simulink model "MARCH_v1_6"  (R2016a)
settings: Solver=FixedStepDiscrete  StartTime=0.0  StopTime=inf  FixedStep=0.001  RelTol=1e-3
InitFcn:
  | cd(fileparts(which(bdroot)));
  | 
  | init_model
  | initialize_model_testingBlocks
StartFcn:
  | cd(fileparts(which(bdroot)));
StopFcn:
  | cd(fileparts(which(bdroot)));
model workspace (MAT data in the model file):
  localValue = 1
  targetValue = 1
undefined symbols (not defined in the file or in its folder): Hip_HAA, Left_Leg, Right_Leg
libraries: xpcethercatlib x56, slrtlib x8, simulink x1, dspnetwork x1, aerolibanimutils x1
(part 2 of 2)

== system MARCH_v1_6/Input Device/Generate random block signal safety/Create peak2 ==
  In1 : Inport
  Delay : Delay  DelayLength=1
  Greater than 0 : MATLAB Function  TreatAsAtomicUnit=on
  Sum : Sum  Inputs=|-+
  Out1 : Outport
  wires:
  Sum/1 -> Greater than 0/1(peak)
  In1/1 -> Sum/2, Delay/1
  Delay/1 -> Sum/1
  Greater than 0/1(signal) -> Out1/1

== system MARCH_v1_6/Input Device/Generate random block signal safety/Create peak3 ==
  In1 : Inport
  Delay : Delay  DelayLength=1
  Greater than 0 : MATLAB Function  TreatAsAtomicUnit=on
  Sum : Sum  Inputs=|-+
  Out1 : Outport
  wires:
  Sum/1 -> Greater than 0/1(peak)
  In1/1 -> Sum/2, Delay/1
  Delay/1 -> Sum/1
  Greater than 0/1(signal) -> Out1/1

== system MARCH_v1_6/Input Device/Generate random block signal trigger/Create peak1 ==
  In1 : Inport
  Delay : Delay  DelayLength=1
  Greater than 0 : MATLAB Function  TreatAsAtomicUnit=on
  Sum : Sum  Inputs=|-+
  Out1 : Outport
  wires:
  Sum/1 -> Greater than 0/1(peak)
  In1/1 -> Sum/2, Delay/1
  Delay/1 -> Sum/1
  Greater than 0/1(signal) -> Out1/1

== system MARCH_v1_6/Input Device/Generate random block signal trigger/Create peak2 ==
  In1 : Inport
  Delay : Delay  DelayLength=1
  Greater than 0 : MATLAB Function  TreatAsAtomicUnit=on
  Sum : Sum  Inputs=|-+
  Out1 : Outport
  wires:
  Sum/1 -> Greater than 0/1(peak)
  In1/1 -> Sum/2, Delay/1
  Delay/1 -> Sum/1
  Greater than 0/1(signal) -> Out1/1

== system MARCH_v1_6/Input Device/Generate random block signal trigger/Create peak3 ==
  In1 : Inport
  Delay : Delay  DelayLength=1
  Greater than 0 : MATLAB Function  TreatAsAtomicUnit=on
  Sum : Sum  Inputs=|-+
  Out1 : Outport
  wires:
  Sum/1 -> Greater than 0/1(peak)
  In1/1 -> Sum/2, Delay/1
  Delay/1 -> Sum/1
  Greater than 0/1(signal) -> Out1/1

== matlab function MARCH_v1_6/Reachability/MATLAB Function ==
  data: q input size=6; q_out output size=6; err output size=6
function [q_out, err] = fcn(q)

joint_limit_min = [-20 -109 -3 -23 -109 -3]'/180*pi;
joint_limit_max = [23 21 121 20 21 121]'/180*pi;

n = size(q,2);
%% Check if all joints are within limits

err = imag(q)~=0 | q<repmat(joint_limit_min,n,1) | q>repmat(joint_limit_max,n,1);
q_out = q;

== matlab function MARCH_v1_6/Controllers/Continuous Gait/Trajectory ==
  data: stepHeight input; q output; done output; stepLength input; q input size=[1 6]; torso_z output; debugIn input; base output; debug output
function [q,done, torso_z, base, debug]= fcn(stepHeight,stepLength,q,debugIn)
%#codegen

persistent r splineCtrl i trajectory fullStep fullWeightShift torsoTrajectory;

%% Initialize all variables
if(isempty(splineCtrl))
    splineCtrl = splineController();
end

if(isempty(fullStep))
    fullStep = 0;
    fullWeightShift = 0;
end

if(isempty(r))
    % Get frequency of the model
    r = robotics();
    r.base = 1;
    
end

if(isempty(i))
    i = 0;
end

if(isempty(trajectory))
    trajectory = [];
    torsoTrajectory = [];
end

%% Logic
% Only run this for the beginning of the swing
r.setTorsoHeight(debugIn);
if(~i)
    
    
    % We set the method of whether we want an analytically generated spline
    % or a spline directly from the database.
    % Options: 'circle' and 'stairs'
    splineCtrl.setStepLength(stepLength).setStepHeight(stepHeight);
    if(~fullStep)
        trajectory = splineCtrl.method('circle').setVelocity(0.7).getHalfStep();
        fullStep = 1;
    else
        trajectory = splineCtrl.method('circle').setVelocity(0.7).getFullStep();
    end
    
    % Transform the spline to the correct frame based on which foot is
    % swinging
    trajectory = r.transformSpline(trajectory);
    
    
    torso_delta = [0 0.1 0];
    
    % Weight shift to base foot
    if(r.base == 1)
        torso_delta(2) = abs(torso_delta(2));
    else
        torso_delta(2) = -abs(torso_delta(2));
    end
    
    if(~fullWeightShift)
        torsoTrajectory = splineCtrl.getHalfWeightShift(torso_delta);
        fullWeightShift = 1;
    else
        torsoTrajectory = splineCtrl.getFullWeightShift(torso_delta);
    end
    
    i = i+1;
end

r.point = [trajectory(1,i) trajectory(2,i) trajectory(3,i)];
debug = r.point;
r.step();
r.weightShift(torsoTrajectory(i,:));

r.inverseKinematics();
q = r.q;

torso_z = r.torso_z;

% Set final values as initial values for the next iteration
r.refresh();

% Reset iterator after we're done with the trajectory, otherwise we
% increment the counter and continue iterating as simulink continues
% sampling
if( i < (length(trajectory)))
    i = i+1;
    done = 0;
else
    i = 0;
    r.switchFoot(r.base);
    done = 1;
end

% Output which foot is currently ON THE GROUND
base = r.base;
end

== matlab function MARCH_v1_6/Controllers/Continuous Gait/Torso Trajectory ==
  data: desired input; current input; z output
function z = fcn(desired, current)
%#codegen

persistent trajectory i desiredPersistent;

% Speed at which we home in SAMPLES
samples = 1000;

if (isempty(i))
    i = 0;
    
    % Hack to fix initial condition of delay during init phase
    current = desired;
end

if(isempty(desiredPersistent))
    desiredPersistent = desired;
end

if(isempty(trajectory))
    trajectory = linspace(current,desiredPersistent,samples);
end

if(desiredPersistent ~= desired)
    trajectory = linspace(current,desired,samples);
    desiredPersistent = desired;
    i = 0;
end

if(i < samples)
    i = i+1;
end

z = trajectory(i);

== matlab function MARCH_v1_6/Controllers/Switcher ==
  data: index output; i input; enable output
function [index, enable]= fcn(i)
%#codegen

% This function is supposed to take a state and switch between controllers.
% Currently it directly routes the input argument as the index. In the
% future this can be something different so I have left it open for
% future modifications.

% The u vector represents the controllers. When the vector consists out of
% zeros it will not enable any controller. In the case that an index is set
% to a non zero value, the controller which belongs to that index will be
% enabled.
u = zeros(10,1);

u(i) = 2;

index = i;
enable = u;

== matlab function MARCH_v1_6/EtherCAT Joint Data In/MATLAB Function ==
  data: encoderValue input; angles output; par parameter
function angles = convertToJointAngles(encoderValue, par)
angles = zeros(6,1);

for i = 1:6
    angles(i) = enc2rad(encoderValue(i), i, par);
end

== matlab function MARCH_v1_6/Controllers/Walking/Trajectory ==
  data: base input; q output; done output; action input; stepType input; q input size=[1 6]
function [q,done]= fcn(base,action,stepType, q)
%#codegen

persistent r splineCtrl i triggerPersistent torsoTrajectory trajectory hold fullWeightShift;

%% Initialize all variables
if(isempty(splineCtrl))
    splineCtrl = splineController();
end

if(isempty(fullWeightShift))
    fullWeightShift = 0;
end

if(isempty(stepType))
    stepType = 0;
end

if(isempty(r))
    % Get frequency of the model
    r = robotics();
    r.base = base;
    
end

if(isempty(hold))
    hold = 0;
end

if(isempty(i))
    i = 0;
end

if(isempty(triggerPersistent))
    triggerPersistent = action;
end


if(isempty(trajectory))
    trajectory = [0 0 0];
    torsoTrajectory = [0 0 0];
end

%% Logic
% Only run this for the beginning of the swing
done = 0;

% Reset values if trigger is toggled.
if(triggerPersistent ~= action)
    r.base = base;
    i = 0;
    hold = 0;
    triggerPersistent = action;
end

% Hold exoskeleton in same position after a single step
if(hold)
    q = r.q;
    done = 1;
    return
end

if(~i)
    % Foot Trajectory
    splineCtrl.setStepHeight(0.5).setStepLength(0.5);
    if(~stepType)
        trajectory = splineCtrl.method('circle').setVelocity(0.5).getHalfStep();
    else
        trajectory = splineCtrl.method('circle').setVelocity(0.5).getFullStep();
    end
    
    trajectory = r.transformSpline(trajectory);
    
    % Weight shift to base foot
    torso_delta = [0 0.07 0];
    
    if(r.base == 1)
        torso_delta(2) = abs(torso_delta(2));
    else
        torso_delta(2) = -abs(torso_delta(2));
    end
    
    if(~stepType)
        torsoTrajectory = splineCtrl.getHalfWeightShift(torso_delta);
    else
        torsoTrajectory = splineCtrl.getFullWeightShift(torso_delta);
    end
    
    
    i = i+1;
end

r.point = [trajectory(1,i) trajectory(2,i) trajectory(3,i)];
r.step();
r.weightShift(torsoTrajectory(i,:));
r.inverseKinematics();

q = r.q;

% Set final values as initial values for the next iteration
r.refresh();

% Reset iterator after we're done with the trajectory, otherwise we
% increment the counter and continue iterating as simulink continues
% sampling
if( i < (length(trajectory)))
    i = i+1;
else
    hold = 1;
end

end

== matlab function MARCH_v1_6/Controllers/Hold/MATLAB Function ==
  data: q_in input size=[1 6]; q_out output double size=[1 6]; reset input
function q_out = fcn(q_in,reset)
persistent q_hold hold

if(isempty(q_hold))
   q_hold = zeros(1,6); 
   hold = 0;
end

if(reset)
   hold = 0; 
end

if(~hold)
    q_hold = q_in;
    hold = 1;
end

q_out = q_hold;

== matlab function MARCH_v1_6/Input Device/Generate random block signal safety/Create peak1/Greater than 0 ==
  data: peak input; signal output
function signal  = fcn(peak)


if peak >= 0
    signal = peak;
else
    signal = 0;
    
    
end

== matlab function MARCH_v1_6/State Machine/Create peak3/Greater than 0 ==
  data: peak input; signal output
function signal  = fcn(peak)


if peak >= 0
    signal = peak;
else
    signal = 0;
    
    
end

== matlab function MARCH_v1_6/Controllers/Point & Go/Trajectory ==
  data: base input; q output; action input; point input; q input size=[1 6]; debugOut output; debugIn input
function [q,debugOut]= fcn(base,action, point,q,debugIn)
%#codegen

persistent r splineCtrl i triggerPersistent trajectory fullStep hold pointPersistent;

%% Initialize all variables
if(isempty(splineCtrl))
    splineCtrl = splineController();
end


if(isempty(fullStep))
    fullStep = 0;
end

if(isempty(r))
    r = robotics();
    r.base = base;
    
end

if(isempty(hold))
    hold = 0;
end

if(isempty(i))
    i = 0;
end

if(isempty(triggerPersistent))
    triggerPersistent = action;
end

if(isempty(pointPersistent))
    pointPersistent = point;
end

if(isempty(trajectory))
    trajectory = [0 0];
end

%% Logic

% Reset values if trigger is toggled.
if(triggerPersistent ~= action)
    r.base = base;
    i = 0;
    hold = 0;
    triggerPersistent = action;
end


% Hold exoskeleton in same position after a single step
if(hold)
    debugOut = r.torso_z;
    q = r.q;
    return
end

if(~i)
    
    % We set the method of whether we want an analytically generated spline
    % or a spline directly from the database.
    % Options: 'circle' and 'stairs'
    splineCtrl.setStepHeight(0.3);
    trajectory = splineCtrl.method('circle').getStepFromPoint(point);
    
    
    
    % Transform the spline to the correct frame based on which foot is
    % swinging
    trajectory = r.transformSpline(trajectory);
    
    i = i+1;
end

r.point = [trajectory(1,i) trajectory(2,i) trajectory(3,i)];

r.stepPosture();
r.inverseKinematics();

q = r.q;
debugOut = r.torso_z;

% Set final values as initial values for the next iteration
r.refresh();

% Reset iterator after we're done with the trajectory, otherwise we
% increment the counter and continue iterating as simulink continues
% sampling
if( i < (length(trajectory)))
    i = i+1;
else
    hold = 1;
end

end

== matlab function MARCH_v1_6/State Machine/Input Interpreter Safety ==
  data: rightIn input; rightOut output; leftIn input; leftOut output; bothOut output
function [rightOut, leftOut, bothOut]= fcn(rightIn, leftIn)

persistent countRight countLeft countBoth

if (isempty(countRight)||isempty(countLeft)||isempty(countBoth));
    countRight = 0;
    countLeft = 0;
    countBoth = 0;
    rightOut = 0;
    leftOut = 0;
    bothOut = 0;
end

threshold = 700;


if (rightIn == 0 && leftIn == 0)
    rightOut = 0;
    leftOut = 0;
    bothOut = 0;
    countRight = 0;
    countLeft = 0;
    countBoth = 0;
elseif (rightIn == 1 && leftIn ~= 1)
    countRight = countRight + 1;
    countLeft = 0;
    countBoth = 0;
    if countRight == threshold
        rightOut = 1;
        leftOut = 0;
        bothOut = 0;
        countRight = 0;
    else
        rightOut = 0;
        leftOut = 0;
        bothOut = 0;
    end
elseif (leftIn == 1 && rightIn ~= 1)
    countRight = 0;
    countLeft = countLeft + 1;
    countBoth = 0;
    if countLeft == threshold
        rightOut = 0;
        leftOut = 1;
        bothOut = 0;
        countLeft = 0;
    else
        rightOut = 0;
        leftOut = 0;
        bothOut = 0;
    end
elseif (rightIn == 1 && leftIn == 1)
    countRight = 0;
    countLeft = 0;
    countBoth = countBoth + 1;
    if countBoth == threshold
        rightOut = 0;
        leftOut = 0;
        bothOut = 1;
    else
        rightOut = 0;
        leftOut = 0;
        bothOut = 0;
    end
else
    rightOut = -1;
    leftOut = -1;
    bothOut = -1;
end

== matlab function MARCH_v1_6/EtherCAT Joint Setpoints/exoskeleton/MATLAB Function ==
  data: jointAngle input; encVal output; par parameter
function encVal = convertToEncoderValues(jointAngle, par)
encVal = zeros(6,1);

for i = 1:6
    encVal(i) = rad2enc(jointAngle(i), i, par);
end

== matlab function MARCH_v1_6/Controllers/StandUp/Trajectory ==
  data: done output; q output; action input; q_i input size=[1 6]; debugIn input
function [done,q] = fcn(action,q_i,debugIn)
%#codegen

persistent r splineCtrl i q_t;

%% Initialize all variables
if(isempty(splineCtrl))
    splineCtrl = splineController();
end

if(isempty(r))
    % Get frequency of the model
    r = robotics();
    
end

if(isempty(q_t))
   q_t = [0 0 0 0 0 0];
end

if(isempty(i))
    i = 0;
end


%% Logic
done = 0;
if(~i)
    % Calculate final position based on robotics parameters
    r.setTorsoHeight(r.torso_z);
    r.refresh();
    r.inverseKinematics();
    q_f = r.q;
    
    splineCtrl.samples = 4000;
    q_t = splineCtrl.getStandupJointTrajectory(q_i,q_f);
    
%     q_t = splineCtrl.ease(q_t);
    
    i = i+1;
end

q = q_t(i,:);

if( i < length(q_t))
    i = i+1;
else
   done = 1; 
end

end

== matlab function MARCH_v1_6/State Machine/Input Interpreter Triggers ==
  data: rightIn input; rightOut output; leftIn input; leftOut output; bothOut output
function [rightOut, leftOut, bothOut]= fcn(rightIn, leftIn)

persistent countRight countLeft countBoth

if (isempty(countRight)||isempty(countLeft)||isempty(countBoth));
    countRight = 0;
    countLeft = 0;
    countBoth = 0;
    rightOut = 0;
    leftOut = 0;
    bothOut = 0;
end

threshold = 700;


if (rightIn == 0 && leftIn == 0)
    rightOut = 0;
    leftOut = 0;
    bothOut = 0;
    countRight = 0;
    countLeft = 0;
    countBoth = 0;
elseif (rightIn == 1 && leftIn ~= 1)
    countRight = countRight + 1;
    countLeft = 0;
    countBoth = 0;
    if countRight == threshold
        rightOut = 1;
        leftOut = 0;
        bothOut = 0;
        countRight = 0;
    else
        rightOut = 0;
        leftOut = 0;
        bothOut = 0;
    end
elseif (leftIn == 1 && rightIn ~= 1)
    countRight = 0;
    countLeft = countLeft + 1;
    countBoth = 0;
    if countLeft == threshold
        rightOut = 0;
        leftOut = 1;
        bothOut = 0;
        countLeft = 0;
    else
        rightOut = 0;
        leftOut = 0;
        bothOut = 0;
    end
elseif (rightIn == 1 && leftIn == 1)
    countRight = 0;
    countLeft = 0;
    countBoth = countBoth + 1;
    if countBoth == threshold
        rightOut = 0;
        leftOut = 0;
        bothOut = 1;
    else
        rightOut = 0;
        leftOut = 0;
        bothOut = 0;
    end
else
    rightOut = -1;
    leftOut = -1;
    bothOut = -1;
end

== matlab function MARCH_v1_6/Controllers/Stairs/Torso Trajectory ==
  data: desired input; torsoTrajectory output size=[1 3]
function torsoTrajectory = fcn(desired)
%#codegen

persistent trajectory i desiredPersistent;

% Speed at which we home in SAMPLES
samples = 1000;

if (isempty(i))
    i = 0;
end

if(isempty(desiredPersistent))
    desiredPersistent = desired;
end

if(isempty(trajectory))   
    desiredPersistent = desired;
    
    trajectory = [linspace(0,desiredPersistent(1),samples)
        linspace(0,desiredPersistent(2),samples)
        linspace(0,desiredPersistent(3),samples) ]';
end

if(~isequal(desiredPersistent,desired))
    trajectory = [linspace(0,desired(1),samples)
        linspace(0,desired(2),samples)
        linspace(0,desired(3),samples) ]';
    
    desiredPersistent = desired;
    i = 0;
end

if(i < samples)
    i = i+1;
end

torsoTrajectory = trajectory(i,:);

== matlab function MARCH_v1_6/Controllers/Stairs/Trajectory ==
  data: base input; q output; action_t input; q input size=[1 6]; torso_delta input size=[1 3]
function q  = fcn(base,action_t,q,torso_delta)
%#codegen

persistent r s i j trigger trajectory torsoTrajectory seq;

%% Initialize all variables
if(isempty(s))
    s = splineController();
end

if(isempty(r))
    % Get frequency of the model
    r = robotics();
    r.base = base;
    
end

if(isempty(seq))
    seq = 1;
end

if(isempty(i) || isempty(j))
    i = 0;
    j = 0;
end

if(isempty(trigger))
    trigger = action_t;
end

if(isempty(torsoTrajectory))
    torsoTrajectory = [0 0 0];
end

if(isempty(trajectory))
    trajectory = [0 0 0];
end

%% Weight shifting sequence
% This sequence will weight shift to the base leg. The entire sequence is
% wrapped inside an if statement to prevent this from executing after it
% has been completed. It is either this or a separate function block which
% would be a disaster because the classes are separate instances.
if(seq == 1)
    if (~i)
        r.setTorsoHeight(0.95);
        r.refresh(); % make sure initial position of torso has same heighit as set above
        % Override sample speed
        s.samples = 1000;
        
        % Weight shift to base foot
        if(base == 1)
            torso_delta(2) = -abs(torso_delta(2));
        else
            torso_delta(2) = abs(torso_delta(2));
        end
        
        torsoTrajectory = s.getHalfWeightShift(torso_delta);
        i = i+1;
    end
    
    % Playback trajectory and return preventing doing the rest
    if(i < length(torsoTrajectory))
        r.reset();
        r.weightShift(torsoTrajectory(i,:));
        r.inverseKinematics();
        q = r.q;
        
        i = i+1;
        return
    else
        q = r.q;
        
        % Init and enable step sequence
        r.refresh();
        j = 0;
        % Disable weight shifting
        seq = 2;
    end
end

%% Step Sequence
% This sequence will step onto the stair
if(seq == 2)
    if(~j)
        s.setStepHeight(0.2).setStepLength(0.5);
        
        trajectory = s.method('circle').setVelocity(0.21).getHalfStep();
        trajectory = r.transformSpline(trajectory);
        if(r.base == 1)
            torso_delta(2) = -abs(torso_delta(2));
        else
            torso_delta(2) = abs(torso_delta(2));
        end
        % Shift the weight back to the middle during the step
        torsoTrajectory = s.getWeightShift(torso_delta, [0 0 0]);
        
        j = j+1;
    end
    
    r.point = [trajectory(1,j) trajectory(2,j) trajectory(3,j)];
    r.step();

    % Weight shift the torso back to the middle
    r.weightShift(torsoTrajectory(j,:));
    r.inverseKinematics();
    
    q = r.q;
    
    % THIS SHOULD NOT BE HERE BUT IT WON'T WORK OTHERWISE :(
    r.refresh();
    
    if(j < length(trajectory))
        j = j+1;
    else
        j = 0;
        q = r.q;
        r.switchFoot(r.base);
    end
    
end
end

== matlab function MARCH_v1_6/Controllers/0-Torque/RHFE/Sample and Hold ==
  data: offset input; reference output
function reference = fcn(offset)
%#codegen

persistent offsetPersistent hold;

if(isempty(offsetPersistent))
    offsetPersistent = int32(0);
    hold = 0;
end

if(offset > 0 && hold == 0)
    
    offsetPersistent = offset;
    hold = 1;
end

reference = offsetPersistent;

== stateflow chart MARCH_v1_6/State Machine/State Machine ==
  state InputDeviceCheck
    en: controllerIndex = 1;
    en: action = 0;
    en: base = 0;
    en: stepType = 0;
    en: state = 0;
    state checkScrollClick
      en: inpDevWorking = 0;
    state checkBothSafety
      en: inpDevWorking = 0;
    state checkbothTrigger
      en: inpDevWorking = 0;
    state InpDev
      en: inpDevWorking = 1;
    (default) -> checkScrollClick : [rightScrollMode == 1]
    checkScrollClick -> checkBothSafety [order 1] : [rightScrollClick == 1]
    checkBothSafety -> checkbothTrigger : [bothSafety == 1]
    checkbothTrigger -> InpDev : [bothTriggers == 1]
  state ZeroTorque
    en: controllerIndex = 1;
    en: action = 0;
    en: base = 0;
    en: stepType = 0;
    en: state = 1;
  state testingBypass
    en: controllerIndex = 1;
    en: action = 0;
    en: base = 0;
    en: stepType = 0;
    en: state = 9;
  state SitDown
    en: controllerIndex = 4;
    en: action = 0;
    en: base = 0;
    en: stepType = 0;
    en: state = 4;
  state HoldPosition
    en: controllerIndex = 2;
    en: action = 0;
    en: base = 0;
    en: stepType = 0;
    en: state = 2;
  state StandUp
    en: controllerIndex = 3;
    en: action = 0;
    en: base = 0;
    en: stepType = 0;
    en: state = 3;
  state DiscreteGait
    en: controllerIndex = 5;
    state standbyModeDiscr
      en: action = actionLocal;
      en: base = baseLocal;
      en: stepType = 0;
      en: state = 61;
      % satandby mode from discrete gait
      % exoskeleton finishes full step, makes complementary halfstep, then stands still
    state makeLeftHalfStepDiscr
      en: action = action+1;
      en: base = 1;
      en: stepType = 0;
      en: state = 61;
      baseLocal = base;
      actionLocal = action;
    state makeRightHalfStepDiscr
      en: action = action+1;
      en: base = 3;
      en: stepType = 0;
      en: state = 61;
      baseLocal = base;
      actionLocal = action;
    state startLeftHalfStepDiscr
      en: action = 1;
      en: base = 1;
      en: stepType = 0;
      en: state = 6;
      baseLocal = base
    state finishRightFullStepDiscr
      en: action = actionLocal;
      en: base = 3;
      en: stepType = 1;
      en: state = 61;
      baseLocal = base;
      % exoskeleton finishes right full step
    state finishLeftFullStepDiscr
      en: action = actionLocal;
      en: base = 1;
      en: stepType = 1;
      en: state = 61;
      baseLocal = base;
      % exoskeleton finishes left full step
    state makeLeftHalfStepDiscr1
      en: action = action+1;
      en: base = 1;
      en: stepType = 0;
      en: state = 62;
      baseLocal = base;
      actionLocal = action;
    state makeRightHalfStepDiscr3
      en: action = action+1;
      en: base = 3;
      en: stepType = 0;
      en: state = 62;
      baseLocal = base;
      actionLocal = action;
    state leftFullStepDiscr
      en: action = action+1;
      en: base = 1;
      en: stepType = 1;
      en: state = 6;
      baseLocal = base;
      actionLocal = action;
    state rightFullStepDiscr
      en: action = action+1;
      en: base = 3;
      en: stepType = 1;
      en: state = 6;
      baseLocal = base;
      actionLocal = action;
    state safeDiscr2Walk1
      en: action = actionLocal;
      en: base = baseLocal;
      en: stepType = 1;
      en: state = 62;
    state safeDiscr2Walk
      en: action = actionLocal;
      en: base = baseLocal;
      en: stepType = 1;
      en: state = 62;
    state safeModeDiscr
      en: action = actionLocal;
      en: base = baseLocal;
      en: stepType = 1;
      en: state = 62;
      % safemode from discr. gait
      % exoskeleton finishes full step, then stands still
    makeRightHalfStepDiscr3 -> standbyModeDiscr : [done == 1]
    makeLeftHalfStepDiscr1 -> standbyModeDiscr : [done == 1]
    standbyModeDiscr -> startLeftHalfStepDiscr [order 2] : [bothTriggers == 1]
    makeLeftHalfStepDiscr -> standbyModeDiscr : [done == 1]
    makeRightHalfStepDiscr -> standbyModeDiscr : [done == 1]
    finishLeftFullStepDiscr -> makeRightHalfStepDiscr : [done == 1]
    finishRightFullStepDiscr -> makeLeftHalfStepDiscr : [done == 1]
    startLeftHalfStepDiscr -> rightFullStepDiscr : [done == 1 && rightTrigger == 1]
    leftFullStepDiscr -> finishLeftFullStepDiscr [order 1] : [bothTriggers == 1]
    rightFullStepDiscr -> finishRightFullStepDiscr [order 1] : [bothTriggers == 1]
    (junction 178) -> makeRightHalfStepDiscr3 [order 2] : [baseLocal == 1]
    (junction 178) -> makeLeftHalfStepDiscr1 [order 1] : [baseLocal == 3]
    rightFullStepDiscr -> leftFullStepDiscr [order 2] : [done == 1 && leftTrigger ==  1]
    leftFullStepDiscr -> rightFullStepDiscr [order 2] : [done == 1 && rightTrigger == 1]
    safeDiscr2Walk1 -> leftFullStepDiscr [order 2] : [leftTrigger == 1 && baseLocal == 3]
    leftFullStepDiscr -> safeModeDiscr [order 3] : [bothSafety == 1]
    rightFullStepDiscr -> safeModeDiscr [order 3] : [bothSafety == 1]
    safeDiscr2Walk1 -> rightFullStepDiscr [order 1] : [rightTrigger == 1 && baseLocal == 1]
    safeDiscr2Walk -> safeDiscr2Walk1 : [done == 1]
    safeModeDiscr -> safeDiscr2Walk [order 1] : [bothSafety == 1]
    safeModeDiscr -> (junction 178) [order 2] : [bothTriggers == 1 && done == 1]
  state ContinuousGait
    en: controllerIndex = 5;
    state standbyModeCont
      en: action = actionLocal;
      en: base = baseLocal;
      en: stepType = 0;
      en: state = 51;
      % satandby mode from continuous gait
      % exoskeleton finishes full step, makes complementary halfstep, then stands still
    state makeLeftHalfStepCont
      en: action = action+1
      en: base = 1;
      en: stepType = 0;
      en: state = 51;
      baseLocal = base;
    state makeRightHalfStepCont
      en: action = action+1;
      en: base = 3;
      en: stepType = 0;
      en: state = 51;
      baseLocal = base;
      actionLocal = action;
    state startLeftHalfStepCont
      en: action = 1;
      en: base = 1;
      en: stepType = 0;
      en: state = 5;
      baseLocal = base
    state finishLeftFullStepCont
      en: action = actionLocal;
      en: base = 1;
      en: stepType = 1;
      en: state = 51;
      baseLocal = base;
      % exoskeleton finishes left full step
    state finishRightFullStepCont
      en: action = actionLocal
      en: base = 3;
      en: stepType = 1;
      en: state = 51;
      baseLocal = base;
      % exoskeleton finishes right full step
    state makeRightHalfStepCont1
      en: action = action+1;
      en: base = 3;
      en: stepType = 0;
      en: state = 52;
      baseLocal = base;
      actionLocal = action;
    state makeLeftHalfStepCont1
      en: action = action+1;
      en: base = 1;
      en: stepType = 0;
      en: state = 52;
      baseLocal = base;
      actionLocal = action
    state leftFullStepCont
      en: action = action+1;
      en: base = 1;
      en: stepType = 1;
      en: state = 5;
      baseLocal = base;
      actionLocal = action;
    state rightFullStepCont
      en: action = action+1
      en: base = 3;
      en: stepType = 1;
      en: state = 5;
      baseLocal = base;
      actionLocal = action;
    state safeCont2Walk
      en: action = actionLocal;
      en: base = baseLocal;
      en: stepType = 1;
      en: state = 52;
    state safeModeCont
      en: action = actionLocal;
      en: base = baseLocal;
      en: stepType = 1;
      en: state = 52;
      % safemode from cont. gait
      % exoskeleton finishes full step, then stands still
    makeRightHalfStepCont1 -> standbyModeCont : [done == 1]
    standbyModeCont -> startLeftHalfStepCont [order 2] : [bothTriggers == 1]
    makeLeftHalfStepCont1 -> standbyModeCont : [done == 1]
    makeRightHalfStepCont -> standbyModeCont : [done == 1]
    makeLeftHalfStepCont -> standbyModeCont : [done == 1]
    finishLeftFullStepCont -> makeRightHalfStepCont : [done == 1]
    finishRightFullStepCont -> makeLeftHalfStepCont : [done == 1]
    startLeftHalfStepCont -> rightFullStepCont : [done == 1]
    leftFullStepCont -> finishLeftFullStepCont [order 2] : [bothTriggers == 1]
    rightFullStepCont -> finishRightFullStepCont [order 1] : [bothTriggers == 1]
    (junction 172) -> makeRightHalfStepCont1 [order 2] : [baseLocal == 1]
    (junction 172) -> makeLeftHalfStepCont1 [order 1] : [baseLocal == 3]
    leftFullStepCont -> rightFullStepCont [order 3] : [done == 1]
    rightFullStepCont -> leftFullStepCont [order 3] : [done == 1]
    safeCont2Walk -> rightFullStepCont [order 1] : [done == 1 && baseLocal == 1]
    rightFullStepCont -> safeModeCont [order 2] : [bothSafety == 1]
    safeCont2Walk -> leftFullStepCont [order 2] : [done == 1 && baseLocal == 3]
    leftFullStepCont -> safeModeCont [order 1] : [bothSafety == 1]
    safeModeCont -> safeCont2Walk [order 1] : [bothSafety == 1]
    safeModeCont -> (junction 172) [order 2] : [bothTriggers == 1 && done == 1]
  (default) -> InputDeviceCheck : [rightScrollMode == 0]
  checkScrollClick -> testingBypass [order 2] : [rightScrollMode == 9]
  InputDeviceCheck -> ZeroTorque : [inpDevWorking == 1]
  ZeroTorque -> HoldPosition : [rightScrollMode == 3 && rightScrollClick == 1]
  SitDown -> ZeroTorque [order 1] : [rightScrollMode == 1 && rightScrollClick == 1 && done == 1]
  HoldPosition -> ZeroTorque [order 1] : [rightScrollMode == 1 && rightScrollClick == 1]
  testingBypass -> StandUp : [rightScrollClick == 1]
  SitDown -> StandUp [order 2] : [rightScrollMode == 3 && rightScrollClick == 1 && done == 1]
  StandUp -> SitDown [order 3] : [rightScrollMode ==4 && rightScrollClick == 1 && done == 1]
  HoldPosition -> StandUp [order 2] : [rightScrollMode == 3 && bothTriggers == 1]
  standbyModeCont -> StandUp [order 1] : [rightScrollMode == 3 && rightScrollClick == 1]
  StandUp -> startLeftHalfStepCont [order 2] : [rightScrollMode == 5 && rightScrollClick == 1 && done == 1]
  StandUp -> startLeftHalfStepDiscr [order 1] : [rightScrollMode == 6 && rightScrollClick == 1 && done == 1]
  standbyModeDiscr -> StandUp [order 1] : [rightScrollMode == 3 && rightScrollClick == 1]
  data: rightTrigger input; leftTrigger input; bothTriggers input; rightSafety input; leftSafety input; bothSafety input; rightScrollMode input; rightScrollClick input; controllerIndex output; action output; base output; inpDevWorking local; done input; stepType output; state output; baseLocal local; actionLocal local

== matlab function MARCH_v1_6/Input Device/Generate random block signal safety/Create peak2/Greater than 0 ==
  data: peak input; signal output
function signal  = fcn(peak)


if peak >= 0
    signal = peak;
else
    signal = 0;
    
    
end

== matlab function MARCH_v1_6/Input Device/Generate random block signal safety/Create peak3/Greater than 0 ==
  data: peak input; signal output
function signal  = fcn(peak)


if peak >= 0
    signal = peak;
else
    signal = 0;
    
    
end

== matlab function MARCH_v1_6/Input Device/Generate random block signal safety/Rand. Block Func. Gen.1 ==
  data: u input; delayDurationInp input; blockDurationInp input; output output
function output  = fcn(u, delayDurationInp, blockDurationInp)

%% initialize the variable
persistent delayDuration blockDuration

if(isempty(blockDuration)||isempty(delayDuration))
    blockDuration = 0;
    delayDuration = 0;
    output = 0;
end

%% check if the delay and the block are done

doneDelay = (delayDuration <= 0);
doneBlock = (blockDuration <= 0);
done = (doneDelay && doneBlock);



%% Create delay and Block

if (u == 0 && done)
    output = 0;
elseif u == 1
    delayDuration = floor(1000*delayDurationInp);
    output = 0;
elseif not(doneDelay)
    delayDuration = delayDuration - 1;
    output = 0;
    if delayDuration == 0
        blockDuration = floor(1000*blockDurationInp);
        output = 1;
    end
elseif not(doneBlock)
    blockDuration = blockDuration - 1;
    output = 1;
else
    output = -1;
end


end

== matlab function MARCH_v1_6/Input Device/Generate random block signal safety/Rand. Block Func. Gen.4 ==
  data: delayDurationInp input; blockDurationInp input; u input; output output
function output  = fcn(delayDurationInp, blockDurationInp, u)

%% initialize the variable
persistent delayDuration blockDuration

if(isempty(blockDuration)||isempty(delayDuration))
    blockDuration = 0;
    delayDuration = 0;
    output = 0;
end



%% check if the delay and the block are done

doneDelay = (delayDuration <= 0);
doneBlock = (blockDuration <= 0);
done = (doneDelay && doneBlock);



%% Create delay and Block

if (u == 0 && done)
    output = 0;
elseif u == 1
    delayDuration = floor(1000*delayDurationInp);
    output = 0;
elseif not(doneDelay)
    delayDuration = delayDuration - 1;
    output = 0;
    if delayDuration == 0
        blockDuration = floor(1000*blockDurationInp);
        output = 1;
    end
elseif not(doneBlock)
    blockDuration = blockDuration - 1;
    output = 1;
else
    output = -1;
end


end

== matlab function MARCH_v1_6/Input Device/Generate random block signal safety/Saturation 2 ==
  data: u input; y output
function y = fcn(u)

min = 0.5;
max = 1.2;

if u <= min
    y = min;
elseif u >= max;
    y = max;
else
    y = u;
end

== matlab function MARCH_v1_6/Input Device/Generate random block signal safety/Saturation1 ==
  data: u input; y output
function y = fcn(u)

min = 0.1;
max = 0.3;

if u <= min
    y = min;
elseif u >= max;
    y = max;
else
    y = u;
end

== matlab function MARCH_v1_6/Input Device/Generate random block signal safety/Saturation3  ==
  data: u input; y output
function y = fcn(u)

min = 0.1;
max = 0.3;

if u <= min
    y = min;
elseif u >= max;
    y = max;
else
    y = u;
end

== matlab function MARCH_v1_6/Input Device/Generate random block signal safety/Saturation4 ==
  data: u input; y output
function y = fcn(u)

min = 0.5;
max = 1.2;

if u <= min
    y = min;
elseif u >= max;
    y = max;
else
    y = u;
end

== matlab function MARCH_v1_6/Input Device/Generate random block signal trigger/Create peak1/Greater than 0 ==
  data: peak input; signal output
function signal  = fcn(peak)


if peak >= 0
    signal = peak;
else
    signal = 0;
    
    
end

== matlab function MARCH_v1_6/Input Device/Generate random block signal trigger/Create peak2/Greater than 0 ==
  data: peak input; signal output
function signal  = fcn(peak)


if peak >= 0
    signal = peak;
else
    signal = 0;
    
    
end

== matlab function MARCH_v1_6/Input Device/Generate random block signal trigger/Create peak3/Greater than 0 ==
  data: peak input; signal output
function signal  = fcn(peak)


if peak >= 0
    signal = peak;
else
    signal = 0;
    
    
end

== matlab function MARCH_v1_6/Input Device/Generate random block signal trigger/Rand. Block Func. Gen.1 ==
  data: u input; delayDurationInp input; blockDurationInp input; output output
function output  = fcn(u, delayDurationInp, blockDurationInp)

%% initialize the variable
persistent delayDuration blockDuration

if(isempty(blockDuration)||isempty(delayDuration))
    blockDuration = 0;
    delayDuration = 0;
    output = 0;
end

%% check if the delay and the block are done

doneDelay = (delayDuration <= 0);
doneBlock = (blockDuration <= 0);
done = (doneDelay && doneBlock);



%% Create delay and Block

if (u == 0 && done)
    output = 0;
elseif u == 1
    delayDuration = floor(1000*delayDurationInp);
    output = 0;
elseif not(doneDelay)
    delayDuration = delayDuration - 1;
    output = 0;
    if delayDuration == 0
        blockDuration = floor(1000*blockDurationInp);
        output = 1;
    end
elseif not(doneBlock)
    blockDuration = blockDuration - 1;
    output = 1;
else
    output = -1;
end


end

== matlab function MARCH_v1_6/Input Device/Generate random block signal trigger/Rand. Block Func. Gen.4 ==
  data: delayDurationInp input; blockDurationInp input; u input; output output
function output   = fcn(delayDurationInp, blockDurationInp, u)

%% initialize the variable
persistent delayDuration blockDuration

if(isempty(blockDuration)||isempty(delayDuration))
    blockDuration = 0;
    delayDuration = 0;
    output = 0;
end



%% check if the delay and the block are done

doneDelay = (delayDuration <= 0);
doneBlock = (blockDuration <= 0);
done = (doneDelay && doneBlock);



%% Create delay and Block

if (u == 0 && done)
    output = 0;
elseif u == 1
    delayDuration = floor(1000*delayDurationInp);
    output = 0;
elseif not(doneDelay)
    delayDuration = delayDuration - 1;
    output = 0;
    if delayDuration == 0
        blockDuration = floor(1000*blockDurationInp);
        output = 1;
    end
elseif not(doneBlock)
    blockDuration = blockDuration - 1;
    output = 1;
else
    output = -1;
end


end

== matlab function MARCH_v1_6/Input Device/Generate random block signal trigger/Saturation 2 ==
  data: u input; y output
function y = fcn(u)

min = 0.5;
max = 1.2;

if u <= min
    y = min;
elseif u >= max;
    y = max;
else
    y = u;
end

== matlab function MARCH_v1_6/Input Device/Generate random block signal trigger/Saturation1 ==
  data: u input; y output
function y = fcn(u)

min = 0.1;
max = 0.3;

if u <= min
    y = min;
elseif u >= max;
    y = max;
else
    y = u;
end

== matlab function MARCH_v1_6/Input Device/Generate random block signal trigger/Saturation3  ==
  data: u input; y output
function y = fcn(u)

min = 0.1;
max = 0.3;

if u <= min
    y = min;
elseif u >= max;
    y = max;
else
    y = u;
end

== matlab function MARCH_v1_6/Input Device/Generate random block signal trigger/Saturation4 ==
  data: u input; y output
function y = fcn(u)

min = 0.5;
max = 1.2;

if u <= min
    y = min;
elseif u >= max;
    y = max;
else
    y = u;
end

== matlab function MARCH_v1_6/Controllers/SitDown/Trajectory ==
  data: q output; action input; q_i input size=[1 6]; debugIn input
function q = fcn(action,q_i,debugIn)
%#codegen

persistent r splineCtrl i q_t;

%% Initialize all variables
if(isempty(splineCtrl))
    splineCtrl = splineController();
end

if(isempty(r))
    % Get frequency of the model
    r = robotics();
    
end

if(isempty(q_t))
   q_t = [0 0 0 0 0 0];
end

if(isempty(i))
    i = 0;
end


%% Logic

if(~i)
    % Calculate final position based on robotics parameters
    r.setTorsoHeight(r.torso_z);
    r.refresh();
    r.inverseKinematics();
    q_f = r.q;
    
    splineCtrl.samples = 4000;
    q_t = splineCtrl.getStandupJointTrajectory(q_i,q_f);
    
    q_t = splineCtrl.ease(q_t);
    
    i = i+1;
end

q = q_t(i,:);

if( i < length(q_t))
    i = i+1;
end

end
